simulink model "Parallel_Dynamic"  (R2015b)
settings: Solver=VariableStepAuto  StartTime=0.0  StopTime=30  RelTol=1e-3
undefined symbols (not defined in the file): A, C, f, g, gear, M, motors, p, R, r, Vw, Zr, Zs
libraries: simulink x1
settings Model: Creator=ihong-gyu  LastModifiedBy=ihong-gyu

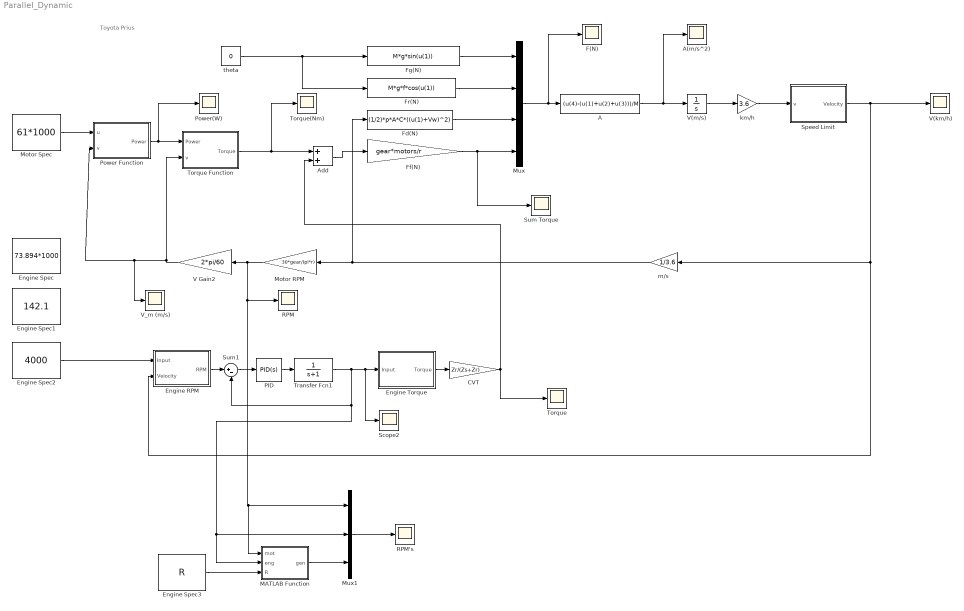
== system Parallel_Dynamic ==
  note: Toyota Prius
  A : Fcn  Expr=(u(4)-(u(1)+u(2)+u(3)))/M
  A(m/s^2) : Scope
  Add : Sum
  CVT : Gain  Gain=Zr/(Zs+Zr)
  Engine RPM : MATLAB Function  TreatAsAtomicUnit=on
  Engine Spec : Constant  Value=73.894*1000
  Engine Spec1 : Constant  Value=142.1
  Engine Spec2 : Constant  Value=4000
  Engine Spec3 : Constant  Value=R
  Engine Torque : MATLAB Function  TreatAsAtomicUnit=on
  F(N) : Scope
  Fd(N) : Fcn  Expr=(1/2)*p*A*C*((u(1)+Vw)^2)
  Ff(N) : Gain  Gain=gear*motors/r
  Fg(N) : Fcn  Expr=M*g*sin(u(1))
  Fr(N) : Fcn  Expr=M*g*f*cos(u(1))
  MATLAB Function : MATLAB Function  TreatAsAtomicUnit=on
  Motor RPM : Gain  Gain=30*gear/(pi*r)
  Motor Spec : Constant  Value=61*1000
  Mux : Mux
  Mux1 : Mux  Inputs=3
  "PID " : simulink/Continuous/PID Controller  Controller=PID  TimeDomain=Continuous-time  SampleTime=-1  IntegratorMethod=Forward Euler  FilterMethod=Forward Euler  Form=Parallel  UseFilter=on  ControllerParametersSource=internal  P=0.665188713135099  I=1.20486835623612  D=0  N=100  InitialConditionSource=internal  InitialConditionForIntegrator=0  InitialConditionForFilter=0  ExternalReset=none  LimitOutput=off  UpperSaturationLimit=inf  LowerSaturationLimit=-inf  LinearizeAsGain=on  AntiWindupMode=none  Kb=1  TrackingMode=off  Kt=1  PParamMin=[]  PParamMax=[]  IParamMin=[]  IParamMax=[]  DParamMin=[]  DParamMax=[]  NParamMin=[]  NParamMax=[]  KbParamMin=[]  KbParamMax=[]  KtParamMin=[]  KtParamMax=[]  POutMin=[]  POutMax=[]  IOutMin=[]  IOutMax=[]  DOutMin=[]  DOutMax=[]  NOutMin=[]  NOutMax=[]  KbOutMin=[]  KbOutMax=[]  KtOutMin=[]  KtOutMax=[]  IntegratorOutMin=[]  IntegratorOutMax=[]  FilterOutMin=[]  FilterOutMax=[]  SumOutMin=[]  SumOutMax=[]  SumI1OutMin=[]  SumI1OutMax=[]  SumI2OutMin=[]  SumI2OutMax=[]  SumI3OutMin=[]  SumI3OutMax=[]  SumDOutMin=[]  SumDOutMax=[]  SaturationOutMin=[]  SaturationOutMax=[]  IntegratorContinuousStateAttributes=''  IntegratorStateMustResolveToSignalObject=off  IntegratorRTWStateStorageClass=Auto  FilterContinuousStateAttributes=''  FilterStateMustResolveToSignalObject=off  FilterRTWStateStorageClass=Auto  DifferentiatorICPrevScaledInput=0  DifferentiatorOutMin=[]  DifferentiatorOutMax=[]
  Power Function : MATLAB Function  TreatAsAtomicUnit=on
  Power(W) : Scope
  RPM : Scope
  RPM's : Scope
  Scope2 : Scope
  Speed Limit : MATLAB Function  TreatAsAtomicUnit=on
  Sum Torque : Scope
  Sum1 : Sum  Inputs=|+-
  Torque : Scope
  "Torque Function " : MATLAB Function  TreatAsAtomicUnit=on
  Torque(Nm) : Scope
  Transfer Fcn1 : TransferFcn  Denominator=[1 1]
  V Gain2 : Gain  Gain=2*pi/60
  V(km/h) : Scope
  V(m/s) : Integrator
  V_m (m/s) : Scope
  km/h : Gain  Gain=3.6
  m/s : Gain  Gain=1/3.6
  theta : Constant  Value=0
  wires:
  Motor Spec/1 -> Power Function/1(u)
  Power Function/1(Power) -> Power(W)/1, "Torque Function "/1(Power)
  Fg(N)/1 -> Mux/1
  Fr(N)/1 -> Mux/2
  Fd(N)/1 -> Mux/3
  Mux/1 -> F(N)/1, A/1
  theta/1 -> Fr(N)/1, Fg(N)/1
  "Torque Function "/1(Torque) -> Add/1, Torque(Nm)/1
  A/1 -> V(m/s)/1, A(m/s^2)/1
  Motor RPM/1 -> MATLAB Function/1(mot), Mux1/1, RPM/1, V Gain2/1
  Ff(N)/1 -> Sum Torque/1, Mux/4
  V Gain2/1 -> "Torque Function "/2(v), V_m (m/s)/1, Power Function/2(v)
  km/h/1 -> Speed Limit/1(v)
  Speed Limit/1(Velocity) -> Engine RPM/2(Velocity), m/s/1, V(km/h)/1
  V(m/s)/1 -> km/h/1
  m/s/1 -> Fd(N)/1, Motor RPM/1
  Engine Spec2/1 -> Engine RPM/1(Input)
  Add/1 -> Ff(N)/1
  Engine Torque/1(Torque) -> CVT/1
  Sum1/1 -> "PID "/1
  "PID "/1 -> Transfer Fcn1/1
  Transfer Fcn1/1 -> MATLAB Function/2(eng), Mux1/2, Sum1/2, Scope2/1, Engine Torque/1(Input)
  Engine RPM/1(RPM) -> Sum1/1
  CVT/1 -> Torque/1, Add/2
  MATLAB Function/1(gen) -> Mux1/3
  Mux1/1 -> RPM's/1
  Engine Spec3/1 -> MATLAB Function/3(R)

== matlab function Parallel_Dynamic/Torque Function  ==
  data: Power input; v input; Torque output
function Torque = fcn(Power, v)
%#codegen

if(Power~=61*1000)
    Torque = 207;
else
    Torque = Power/v;
end

== matlab function Parallel_Dynamic/Power Function ==
  data: u input; Power output; v input
function Power = fcn(u, v)
%#codegen

if(v~=0)
    Power=v*207;
else
    Power=1;
end

if(Power>61*1000)
    Power=61*1000;
end

== matlab function Parallel_Dynamic/Speed Limit ==
  data: v input; Velocity output
function Velocity = fcn(v)
%#codegen

if(v>154)
    Velocity=154;
else
    Velocity=v;
end

== matlab function Parallel_Dynamic/Engine RPM ==
  data: Input input; RPM output; Velocity input
function RPM = fcn(Input, Velocity)
%#codegen

if(Velocity<30)
    RPM=0;
else
    RPM=Input;
end

== matlab function Parallel_Dynamic/Engine Torque ==
  data: Input input; Torque output
function Torque = fcn(Input)
%#codegen

if(Input~=0)
    Torque=142.1*Input/4000;
else
    Torque=0;
end

== matlab function Parallel_Dynamic/MATLAB Function ==
  data: mot input; gen output; eng input; R input
function gen = fcn(mot, eng, R)
%#codegen

gen = ((1+R)*eng-mot)/R;
